simulink model "sailboat_ap_ok"  (Simulink 8.3)
settings: Solver=FixedStepDiscrete  StartTime=0.0  StopTime=1000  FixedStep=0.1  RelTol=1e-3
model workspace: external: MATLAB File (data not in the file)
undefined symbols (not defined in the file): DiscIntNeverNeededParam, rudderD, rudderI, rudderP, sailD, sailI, sailP
libraries: simulink x2
settings Model: Creator=建云  LastModifiedBy=edison  NumberOfSteps=5  TunableVars=kp,wind  TunableVarsStorageClass=Auto,Auto  TunableVarsTypeQualifier=,
settings DataIOCC: SignalLoggingSaveFormat=Dataset
settings OptimizationCC: OptimizeModelRefInitCode=on  LifeSpan=1
settings DebuggingCC: FrameProcessingCompatibilityMsg=error  StateNameClashWarn=none
settings HardwareCC: ProdBitPerLong=64  ProdBitPerPointer=64  ProdLargestAtomicFloat=Float  ProdIntDivRoundTo=Zero  ProdEndianess=LittleEndian  ProdWordSize=64  ProdHWDeviceType=Intel->x86-64 (Linux 64)
settings RTWCC: SystemTargetFile=ert.tlc  GenCodeOnly=on  TemplateMakefile=ert_default_tmf  Description=Embedded Coder  GenerateReport=on  ProcessScript=ert_make_rtw_hook  Toolchain=Microsoft Windows SDK v7.1 | nmake (32-bit Windows)  IncludeHyperlinkInReport=on  LaunchReport=on  TargetLang=C++  GenerateTraceInfo=on  GenerateTraceReport=on  GenerateTraceReportSl=on  GenerateTraceReportSf=on  GenerateTraceReportEml=on
settings CodeAppCC: ForceParamTrailComments=on  SimulinkDataObjDesc=on  CustomSymbolStrGlobalVar=rt$N$M  CustomSymbolStrType=$N$M  CustomSymbolStrFcn=$N$M$F  CustomSymbolStrMacro=$N$M  InsertBlockDesc=on
settings ERTTargetCC: TargetLangStandard=C++03 (ISO)  MultiwordLength=2048  GenerateSampleERTMain=on  MultiInstanceERTCode=on  CodeInterfacePackaging=C++ class  SupportVariableSizeSignals=on  RootIOFormat=Structure reference  ERTCustomFileTemplate=example_file_process.tlc  ERTFilePackagingFormat=CompactWithDataFile  ConvertIfToSwitch=off  SuppressUnreachableDefaultCases=off
settings CPPComponent: GenerateDestructor=on  GenerateExternalIOAccessMethods=None  ParameterMemberVisibility=public  InternalMemberVisibility=public  GenerateParameterAccessMethods=None  GenerateInternalMemberAccessMethods=None  UseOperatorNewForModelRefRegistration=off
settings ConfigComp: CovMetricSettings=dw  CovHtmlReporting=on  CovSaveCumulativeToWorkspaceVar=on  CovSaveSingleToWorkspaceVar=on  CovExternalEMLEnable=off

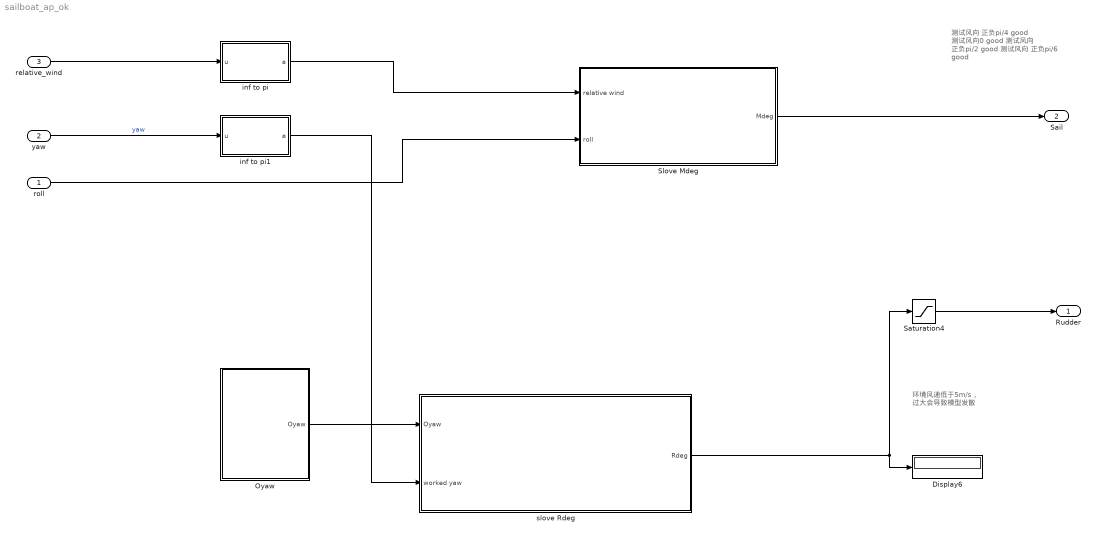
== system sailboat_ap_ok ==
  note: 环境风速低于5m/s，
      | 过大会导致模型发散
  note: 测试风向 正负pi/4 good
      | 测试风向0 good
      | 测试风向 正负pi/2 good
      | 测试风向 正负pi/6 good
  roll : Inport
  yaw : Inport  Port=2
  relative_wind : Inport  Port=3
  " Slove Mdeg" : Subsystem  TreatAsAtomicUnit=on
  Display6 : Display
  Oyaw : MATLAB Function  TreatAsAtomicUnit=on
  Saturation4 : Saturate  UpperLimit=0.68  LowerLimit=-0.68
  inf to pi : MATLAB Function  TreatAsAtomicUnit=on
  inf to pi1 : MATLAB Function  TreatAsAtomicUnit=on
  slove Rdeg : Subsystem  TreatAsAtomicUnit=on
  Rudder : Outport
  Sail : Outport  Port=2
  wires:
  inf to pi1/1(a) -> slove Rdeg/2(worked yaw)
  yaw/1 -> inf to pi1/1(u)  "yaw"
  roll/1 -> " Slove Mdeg"/2(roll)
  slove Rdeg/1(Rdeg) -> Saturation4/1, Display6/1
  inf to pi/1(a) -> " Slove Mdeg"/1(relative wind)
  " Slove Mdeg"/1(Mdeg) -> Sail/1
  Saturation4/1 -> Rudder/1
  relative_wind/1 -> inf to pi/1(u)
  Oyaw/1(Oyaw) -> slove Rdeg/1(Oyaw)

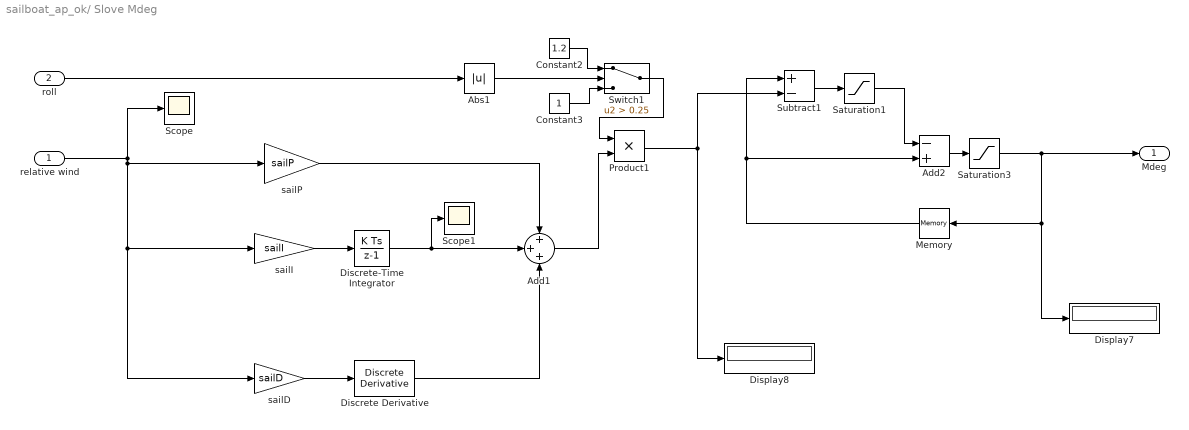
== system sailboat_ap_ok/ Slove Mdeg ==
  relative wind : Inport
  roll : Inport  Port=2
  Abs1 : Abs
  Add1 : Sum  Inputs=+++
  Add2 : Sum  Inputs=-+
  Constant2 : Constant  Value=1.2
  Constant3 : Constant
  Discrete Derivative : simulink/Discrete/Discrete Derivative  gainval=1.0  ICPrevScaledInput=0.0  InputProcessing=Inherited  OutMin=[]  OutMax=[]  OutDataType=fixdt(1, 16)  OutScaling=2^-10  DoSatur=off
  Discrete-Time Integrator : DiscreteIntegrator  InitialConditionSetting=State (most efficient)  SampleTime=-1  ICPrevOutput=DiscIntNeverNeededParam  ICPrevScaledInput=DiscIntNeverNeededParam
  Display7 : Display
  Display8 : Display
  Memory : Memory
  Product1 : Product
  Saturation1 : Saturate  UpperLimit=0.20  LowerLimit=-0.20
  Saturation3 : Saturate  UpperLimit=1.39  LowerLimit=-1.39
  Scope : Scope
      settings: YMin=0  YMax=2.5  SaveName=ScopeData8
  Scope1 : Scope
      settings: YMin=0.0005  YMax=0.0009  SaveName=ScopeData9
  Subtract1 : Sum  Inputs=+-
  Switch1 : Switch  Criteria=u2 > Threshold  Threshold=0.25
  sailD : Gain  Gain=sailD
  sailI : Gain  Gain=sailI
  sailP : Gain  Gain=sailP
  Mdeg : Outport
  wires:
  Subtract1/1 -> Saturation1/1
  Saturation1/1 -> Add2/1
  Memory/1 -> Subtract1/1, Add2/2
  Product1/1 -> Subtract1/2, Display8/1
  Constant3/1 -> Switch1/3
  Constant2/1 -> Switch1/1
  Add1/1 -> Product1/2
  Switch1/1 -> Product1/1
  Abs1/1 -> Switch1/2
  Saturation3/1 -> Memory/1, Display7/1, Mdeg/1
  roll/1 -> Abs1/1
  Add2/1 -> Saturation3/1
  sailI/1 -> Discrete-Time Integrator/1
  sailD/1 -> Discrete Derivative/1
  relative wind/1 -> sailD/1, sailI/1, sailP/1, Scope/1
  sailP/1 -> Add1/1
  Discrete-Time Integrator/1 -> Scope1/1, Add1/2
  Discrete Derivative/1 -> Add1/3

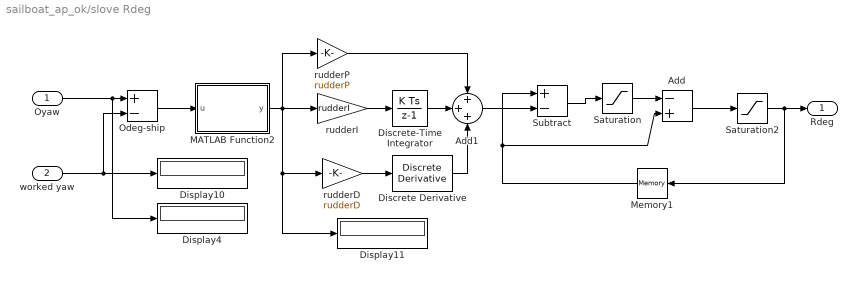
== system sailboat_ap_ok/slove Rdeg ==
  Oyaw : Inport
  worked yaw : Inport  Port=2
  Add : Sum  Inputs=-+
  Add1 : Sum  Inputs=+++
  Discrete Derivative : simulink/Discrete/Discrete Derivative  gainval=1.0  ICPrevScaledInput=0.0  InputProcessing=Inherited  OutMin=[]  OutMax=[]  OutDataType=fixdt(1, 16)  OutScaling=2^-10  DoSatur=off
  Discrete-Time Integrator : DiscreteIntegrator  InitialConditionSetting=State (most efficient)  SampleTime=-1  ICPrevOutput=DiscIntNeverNeededParam  ICPrevScaledInput=DiscIntNeverNeededParam
  Display10 : Display
  Display11 : Display
  Display4 : Display
  MATLAB Function2 : MATLAB Function  TreatAsAtomicUnit=on
  Memory1 : Memory
  Odeg-ship : Sum  Inputs=+-
  Saturation : Saturate  UpperLimit=0.175  LowerLimit=-0.175
  Saturation2 : Saturate  UpperLimit=0.68  LowerLimit=-0.68
  Subtract : Sum  Inputs=+-
  rudderD : Gain  Gain=rudderD
  rudderI : Gain  Gain=rudderI
  rudderP : Gain  Gain=rudderP
  Rdeg : Outport
  wires:
  Oyaw/1 -> Display4/1, Odeg-ship/1
  Subtract/1 -> Saturation/1
  Saturation/1 -> Add/1
  Add1/1 -> Subtract/2
  Memory1/1 -> Subtract/1, Add/2
  Odeg-ship/1 -> MATLAB Function2/1(u)
  worked yaw/1 -> Odeg-ship/2, Display10/1
  Add/1 -> Saturation2/1
  Saturation2/1 -> Memory1/1, Rdeg/1
  rudderI/1 -> Discrete-Time Integrator/1
  rudderD/1 -> Discrete Derivative/1
  MATLAB Function2/1(y) -> rudderD/1, Display11/1, rudderI/1, rudderP/1
  rudderP/1 -> Add1/1
  Discrete-Time Integrator/1 -> Add1/2
  Discrete Derivative/1 -> Add1/3

== matlab function inf to pi ==
  data: a output double; u input double
function a  = fcn(u)
%#chushihua
while abs(u)>pi
    if u>pi
        u = u-2*pi;
    elseif u<-pi
        u = u+2*pi;
    end
end       
a = u;

== matlab function inf to pi1 ==
  data: a output double; u input double
function a  = fcn(u)
%#chushihua
while abs(u)>pi
    if u>pi
        u = u-2*pi;
    elseif u<-pi
        u = u+2*pi;
    end
end       
a = u;

== matlab function Oyaw ==
  data: Oyaw output double; oyaw parameter double
function Oyaw  = fcn(oyaw)
Oyaw = oyaw;

== matlab function slove Rdeg/MATLAB Function2 ==
  data: u input double; y output double
function y = fcn(u)
%#codegen
if u>pi
    y = u-2*pi;
elseif u<-pi
    y = u+2*pi;
else
    y=u;
end
